simulink library "ctg"  (Simulink 8.1)
settings: Solver=ode1  StartTime=0.0  StopTime=Inf  FixedStep=0.001  RelTol=1e-3
PostLoadFcn:
  | , if any(exist('dsrtsu_mdlpostloadfcn', 'file') == [2, 3, 6]), try dsrtsu_mdlpostloadfcn('Execute', bdroot); catch fprintf('Error in PostLoadFcn (dsrtsu_mdlpostloadfcn) for model "%s":\n %s\n', bdroot, lasterr); end, end,
undefined symbols (not defined in the file or in its folder): KACC_ACCTqReleaseFixedMargin_flg, KACC_ACCTqReleaseMargin_m, KACC_ACCTransitionSlope_num, KACC_ConsideredSetTimeGap_s, KACC_ReleaseTGapPerc_perc
settings Model: DSRTSU_INTERNAL_RTI_VER=450  DSRTSU_INTERNAL_RTI_TYPE=rti1401  RTICANMMDATA=struct('GeneralSetupData',struct('modelroot','C:\Users\idiada\Desktop\HAITEC_Taiwan\trunk\AdasDragon\software\sw_development\arch\app\acc','generalsettings',struct('filesettings',struct('destfolder',struct('Name','RTICANMM_FILES','Check',1),'buildfolder',struct('Name','.','Check',1),'AbsDestfolder',struct('Name','C:\Users\idiada\Desktop\HAITEC_Taiwan\trunk\AdasDragon\software\sw_development\arch\app\acc\RTICANMM_FILES'),'AbsBuildfolder',struct('Name','C:\Users\idiada\Desktop\HAITEC_Taiwan\trunk\AdasDragon\software\sw_development\arch\app\acc'))),'options',struct('addpaths',1,'rmpaths',1,'addtrcexclusion',logical(1),'cannavigator',struct('checkmonitoring',0),'show_usrtrc',0,'use_usrtrc',0),'advanced',struct('options',[1 1 1 1 1 1 1 1 1 1 1 1 1 1 1 1 1 1 1 1 1 1 1 1 1 1 1 1 1 1 1 1 1 1 1 1 1 1 1 1 1 1 1 1 1 1 1 1 1 1 1 1 1 1 1 1 1 1 1 1 1 1 1 1 1 1 1 1 1 1 1 1 1 1 1 1 1 1 1 1 1 1 1 1 1 1 1 1 1 1 1 1 1 1 1 1 1 1 1 1]),'MPSetup',{{}},'modelname','ctg','block','ctg'))  DSRTSU_INTERNAL_RTIFPGA=40  Creator=idiada  LastModifiedBy=idiada

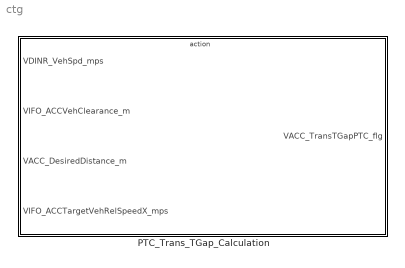
== system ctg ==
  PTC_Trans_TGap_Calculation : Subsystem  TreatAsAtomicUnit=on

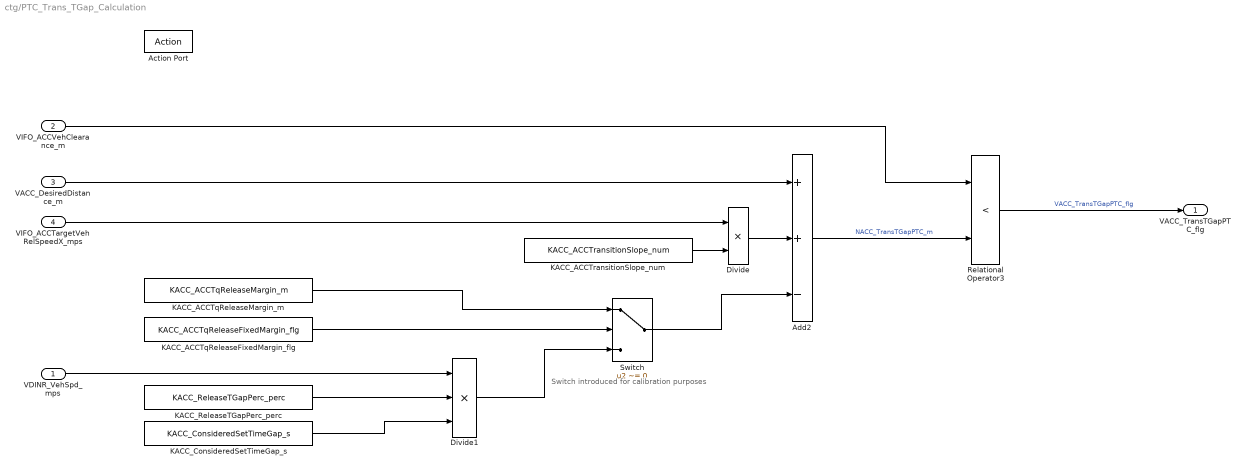
== system ctg/PTC_Trans_TGap_Calculation ==
  note: Switch introduced for calibration purposes
  VDINR_VehSpd_mps : Inport
  VIFO_ACCVehClearance_m : Inport  Port=2
  VACC_DesiredDistance_m : Inport  Port=3
  VIFO_ACCTargetVehRelSpeedX_mps : Inport  Port=4
  Action Port : ActionPort
  Add2 : Sum  Inputs=++-
  Divide : Product  Inputs=**
  Divide1 : Product  Inputs=***
  KACC_ACCTqReleaseFixedMargin_flg : Constant  Value=KACC_ACCTqReleaseFixedMargin_flg
  KACC_ACCTqReleaseMargin_m : Constant  Value=KACC_ACCTqReleaseMargin_m
  KACC_ACCTransitionSlope_num : Constant  Value=KACC_ACCTransitionSlope_num
  KACC_ConsideredSetTimeGap_s : Constant  Value=KACC_ConsideredSetTimeGap_s
  KACC_ReleaseTGapPerc_perc : Constant  Value=KACC_ReleaseTGapPerc_perc
  Relational Operator3 : RelationalOperator  Operator=<  OutDataTypeStr=boolean
  Switch : Switch  Criteria=u2 ~= 0
  VACC_TransTGapPTC_flg : Outport
  wires:
  Switch/1 -> Add2/3
  KACC_ACCTqReleaseMargin_m/1 -> Switch/1
  KACC_ACCTqReleaseFixedMargin_flg/1 -> Switch/2
  KACC_ConsideredSetTimeGap_s/1 -> Divide1/3
  KACC_ReleaseTGapPerc_perc/1 -> Divide1/2
  VDINR_VehSpd_mps/1 -> Divide1/1
  Divide1/1 -> Switch/3
  Relational Operator3/1 -> VACC_TransTGapPTC_flg/1  "VACC_TransTGapPTC_flg"
  VIFO_ACCVehClearance_m/1 -> Relational Operator3/1
  VIFO_ACCTargetVehRelSpeedX_mps/1 -> Divide/1
  VACC_DesiredDistance_m/1 -> Add2/1
  KACC_ACCTransitionSlope_num/1 -> Divide/2
  Add2/1 -> Relational Operator3/2  "NACC_TransTGapPTC_m"
  Divide/1 -> Add2/2
